simulink model "Experimental_estimation_Kphi_B_tau_s"  (R2022b)
settings: Solver=VariableStepAuto  StartTime=0.0  StopTime=10.0  RelTol=1e-3
undefined symbols (not defined in the file or in its folder): Hi, Hw, sens
libraries: arduinolib x5, simulink x1
settings Model: Creator=berti  LastModifiedBy=berti

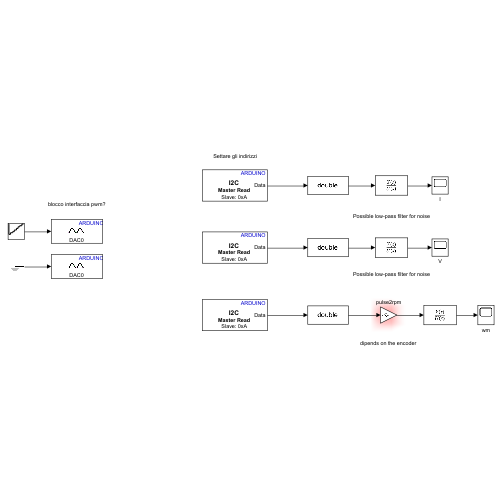
[thumbnail: Simulink's stored preview of the top-level diagram]
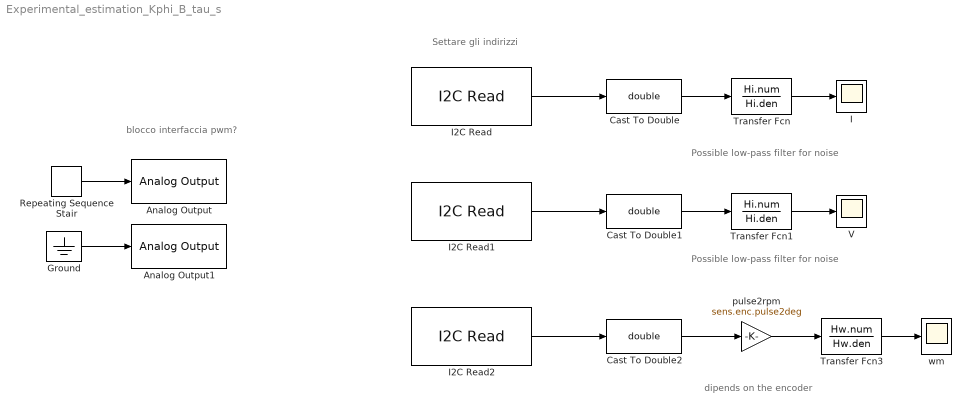
== system Experimental_estimation_Kphi_B_tau_s ==
  note: blocco interfaccia pwm?
  note: Settare gli indirizzi
  note: dipends on the encoder
  note: Possible low-pass filter for noise
  note: Possible low-pass filter for noise
  Analog Output : arduinolib/Analog Output  DACpin=DAC0  blockPlatform=arduino
  Analog Output1 : arduinolib/Analog Output  DACpin=DAC0  blockPlatform=arduino
  Cast To Double : DataTypeConversion  OutDataTypeStr=double  SaturateOnIntegerOverflow=off  RndMeth=Floor
  Cast To Double1 : DataTypeConversion  OutDataTypeStr=double  SaturateOnIntegerOverflow=off  RndMeth=Floor
  Cast To Double2 : DataTypeConversion  OutDataTypeStr=double  SaturateOnIntegerOverflow=off  RndMeth=Floor
  Ground : Ground
  I : Scope
  I2C Read : arduinolib/I2C Read  I2CModule=0  Mode=Master  SlaveAddress=10  SlaveByteOrder=BigEndian  Direction=Receiver  RegisterAddressMode=on  RegisterAddress=0  SlaveDataType=uint8  DataLength=1  NoAck=off  RepeatedStart=off  OutputStatus=off  blockPlatform=ARDUINO  SampleTime=0.1
  I2C Read1 : arduinolib/I2C Read  I2CModule=0  Mode=Master  SlaveAddress=10  SlaveByteOrder=BigEndian  Direction=Receiver  RegisterAddressMode=on  RegisterAddress=0  SlaveDataType=uint8  DataLength=1  NoAck=off  RepeatedStart=off  OutputStatus=off  blockPlatform=ARDUINO  SampleTime=0.1
  I2C Read2 : arduinolib/I2C Read  I2CModule=0  Mode=Master  SlaveAddress=10  SlaveByteOrder=BigEndian  Direction=Receiver  RegisterAddressMode=on  RegisterAddress=0  SlaveDataType=uint8  DataLength=1  NoAck=off  RepeatedStart=off  OutputStatus=off  blockPlatform=ARDUINO  SampleTime=0.1
  Repeating Sequence Stair : simulink/Sources/Repeating Sequence Stair  OutValues=0.5*[1 2 3 4 5 6 7 8].'  tsamp=5  OutMin=[]  OutMax=[]  OutDataTypeStr=double  OutputDataTypeScalingMode=double  OutDataType=fixdt(0,8)  ConRadixGroup=Best Precision: Vector-wise  OutScaling=2^-12
  Transfer Fcn : TransferFcn  Numerator=Hi.num  Denominator=Hi.den
  Transfer Fcn1 : TransferFcn  Numerator=Hi.num  Denominator=Hi.den
  Transfer Fcn3 : TransferFcn  Numerator=Hw.num  Denominator=Hw.den
  V : Scope
  pulse2rpm : Gain  Gain=sens.enc.pulse2deg
  wm : Scope
  wires:
  Repeating Sequence Stair/1 -> Analog Output/1
  Transfer Fcn/1 -> I/1
  pulse2rpm/1 -> Transfer Fcn3/1
  Cast To Double/1 -> Transfer Fcn/1
  Cast To Double2/1 -> pulse2rpm/1
  Cast To Double1/1 -> Transfer Fcn1/1
  Transfer Fcn1/1 -> V/1
  Transfer Fcn3/1 -> wm/1
  I2C Read/1 -> Cast To Double/1
  I2C Read1/1 -> Cast To Double1/1
  I2C Read2/1 -> Cast To Double2/1
  Ground/1 -> Analog Output1/1
